simulink model "combined_model_withAC_2021b"  (R2021b)
settings: Solver=VariableStepAuto  StartTime=0.0  StopTime=5  RelTol=1e-3
model workspace (MAT data in the model file):
  C = 0.00044
  L = 0.00025
undefined symbols (not defined in the file): C_phi, Ls, poles, powergui, R_load, Rs, spspowerguiLib
libraries: spsDiodeLib x7, spsSeriesRLCBranchLib x6, spsVoltageMeasurementLib x5, spsMosfetLib x5, spsControlledVoltageSourceLib x3, simulink x3, spsCurrentMeasurementLib x2, spsParallelRLCBranchLib x2, spsGroundLib x1, spsParallelRLCLoadLib x1, spsVariableCapacitorLib x1
settings Model: Creator=maarten  LastModifiedBy=maarten
settings DebuggingCC: UnconnectedInputMsg=none  UnconnectedOutputMsg=none  UnconnectedLineMsg=none
settings ModelReferenceCC: EnableRefExpFcnMdlSchedulingChecks=off
settings RTWCC: DLArmComputeVersion=20.02.1

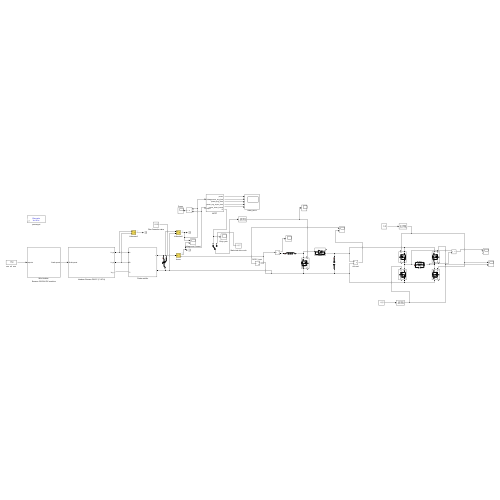
[thumbnail: Simulink's stored preview of the top-level diagram]
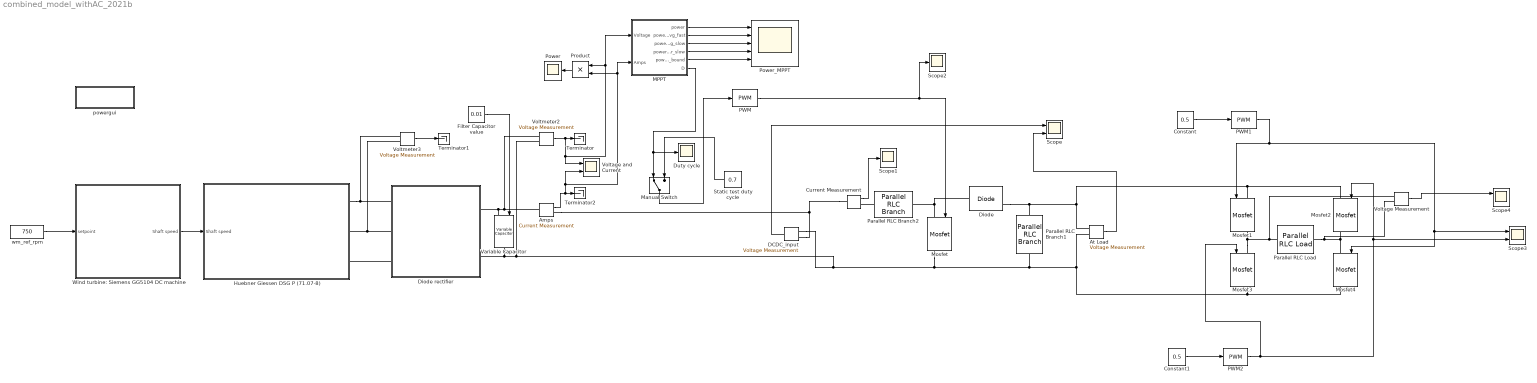
== system combined_model_withAC_2021b ==
  Amps : spsCurrentMeasurementLib/Current Measurement  PhasorSimulation=off  OutputType=Complex  PSBequivalent=0
  At Load : spsVoltageMeasurementLib/Voltage Measurement  PhasorSimulation=off  OutputType=Complex  PSBequivalent=0
  Constant : Constant  Value=0.5
  Constant1 : Constant  Value=0.5
  Current Measurement : spsCurrentMeasurementLib/Current Measurement  PhasorSimulation=off  OutputType=Complex  PSBequivalent=0
  DCDC_input : spsVoltageMeasurementLib/Voltage Measurement  PhasorSimulation=off  OutputType=Complex  PSBequivalent=0
  Diode : spsDiodeLib/Diode  Ron=0.001  Lon=0  Vf=0.8  IC=0  UseSnubber=0  Rs=500  Cs=250e-9  Measurements=on
  Diode rectifier : Subsystem
  Duty cycle : Scope
  Filter Capacitor value : Constant  Value=0.01
  "Huebner Giessen DSG P (71.07-8) " : Subsystem
  MPPT : Subsystem
  Manual Switch : ManualSwitch
  Mosfet{,1..4} (5 alike) : spsMosfetLib/Mosfet  Ron=0.1  Lon=0  Rd=0.01  Vfd=0  IC=0  Rs=1e5  Cs=inf  Measurements=on
  PWM : simulink/Discontinuities/PWM  DisableCoverage=on  Period=0.0001  InitialDelay=0  DisallowZeroDutyCycle=off  RunAtFixedTimeIntervals=off  SampleTime=0.1
  PWM1 : simulink/Discontinuities/PWM  DisableCoverage=on  Period=0.0005  InitialDelay=0  DisallowZeroDutyCycle=off  RunAtFixedTimeIntervals=off  SampleTime=0.1
  PWM2 : simulink/Discontinuities/PWM  DisableCoverage=on  Period=0.0005  InitialDelay=0.0005/2  DisallowZeroDutyCycle=off  RunAtFixedTimeIntervals=off  SampleTime=0.1
  Parallel RLC Branch1 : spsParallelRLCBranchLib/Parallel RLC Branch  LConnTagsString=a  RConnTagsString=__new0  BranchType=C  Resistance=R_load  Inductance=1e-3  SetiL0=off  InitialCurrent=0  Capacitance=C  Setx0=off  InitialVoltage=0  Measurements=None
  Parallel RLC Branch2 : spsParallelRLCBranchLib/Parallel RLC Branch  LConnTagsString=a  RConnTagsString=__new0  BranchType=L  Resistance=R_load  Inductance=L  SetiL0=off  InitialCurrent=0  Capacitance=C  Setx0=off  InitialVoltage=0  Measurements=None
  Parallel RLC Load : spsParallelRLCLoadLib/Parallel RLC Load  LConnTagsString=a  RConnTagsString=__new0  NominalVoltage=1000  NominalFrequency=60  ActivePower=10e3  InductivePower=100  CapacitivePower=100  Setx0=off  InitialVoltage=0  SetiL0=off  InitialCurrent=0  Measurements=None  LoadType=constant Z
      settings: AttributesFormatString=\n
  Power : Scope
  Power_MPPT : Scope  NumInputPorts=5
  Product : Product
  Scope : Scope  NumInputPorts=2
  Scope1 : Scope
  Scope2 : Scope
  Scope3 : Scope  NumInputPorts=2
  Scope4 : Scope  NumInputPorts=2
  Static test duty cycle : Constant  Value=0.7
  Terminator : Terminator
  Terminator1 : Terminator
  Terminator2 : Terminator
  Variable Capacitor : spsVariableCapacitorLib/Variable Capacitor  methode=Backward Euler  Cabsmin=1e-9  Initialize=off  vC0=0  C0=1e-6  iC0=0
  Voltage Measurement : spsVoltageMeasurementLib/Voltage Measurement  PhasorSimulation=off  OutputType=Complex  PSBequivalent=0
  Voltage and Current : Scope  NumInputPorts=2
  Voltmeter2 : spsVoltageMeasurementLib/Voltage Measurement  PhasorSimulation=off  OutputType=Complex  PSBequivalent=0
  Voltmeter3 : spsVoltageMeasurementLib/Voltage Measurement  PhasorSimulation=off  OutputType=Complex  PSBequivalent=0
  "Wind turbine: Siemens GG5104 DC machine " : Subsystem
  powergui : Subsystem  Priority=1  AncestorBlock=spspowerguiLib/powergui  DialogController=POWERSYS.PowerSysDialog  InitFcn=powergui( 'InitFcn_Callback' , gcb , 0 , [ ] );  mask(PSB option menu block){SimulationMode=Discrete, SampleTime=1e-6, frequency=60, Iterations=50, frequencyindice=0, Pbase=100e6, ErrMax=1e-4, UnitsV=kV, UnitsW=MW, buscounter=0, FunctionMessages=off, echomessages=off, EnableUseOfTLC=off, CurrentSourceSwitches=off, DisableSnubberDevices=off, DisableRonSwitches=off, DisableVfSwitches=off, DisplayEquations=off, AutomaticDiscreteSolvers=off, SolverType=Tustin, Interpol=off, ExternalGateDelay=off, methode=off, Ts=0, x0status=blocks, SPID=off, SwTol=0, HookPort=off, NonlinearTolerance=1e-4, nMaxIteration=100, ContinueOnMaxIteration=off, RestoreLinks=warning, ResistiveCurrentMeasurement=off, Frange=[0:2:500], Ylog=off, Xlog=on, ShowGrid=off, save=off, variable=ZData, structure=0, ZoomFFT=off, StartTime=0.0, cycles=1, DisplayStyle=1, fundamental=60, FreqAxis=off, MaxFrequency=1000, frequencyindicesteady=1, RmsSteady=1, display=off}
      mask prompts: SimulationMode "Simulation type:"; SampleTime "Sample time (s):"; frequency "Frequency (Hz):"; Iterations "Max iterations"; frequencyindice "Frequency (Hz)"; Pbase "Base power (VA)"; ErrMax "PQ tolerance (pu)"; UnitsV "Voltage units"; UnitsW "Power units"; buscounter "Load flow bus counter"; FunctionMessages "Disable Specialized Power Systems warnings"; echomessages "Display Specialized Power Systems compilation messages"; EnableUseOfTLC "Use TLC file when in Accelerator Simulation Mode and for code generation"; CurrentSourceSwitches "Disable ideal switching"; DisableSnubberDevices "Disable snubbers in switching devices"; DisableRonSwitches "Disable Ron resistances in switching devices"; DisableVfSwitches "Disable forward voltages in switching devices"; DisplayEquations "Display circuit differential equations"; AutomaticDiscreteSolvers "Automatically handle Discrete solver and Advanced tab solver settings of blocks"; SolverType "Discrete solver"; Interpol "Interpolate switching events"; ExternalGateDelay "Use time-stamped gate signals"; methode "Store switching topologies"; Ts "Buffer size (MBytes):"; x0status "Start simulation with initial electrical states from:"; SPID "Use ideal switching devices"; SwTol "Switch tolerance"; HookPort "Allow multiple powergui blocks"; NonlinearTolerance "Solver tolerance"; nMaxIteration "Maximum number of iterations"; ContinueOnMaxIteration "Continue Simulation if maximum number of iterations is reached"; RestoreLinks "Restore disabled links of Simscape Power Systems ST blocks:"; ResistiveCurrentMeasurement "Use non ideal current measurement blocks (1e-4Ohm internal resistance)"; Frange "Frequency Range"; Ylog "Log impedance"; Xlog "log Frequency"; ShowGrid "grid"; save "Save Data To Workspace"; variable "Variable Name"; structure "Structure Name (PSBFFTSCOPE)"; ZoomFFT "ZoomFFT (PSBFFTSCOPE)"; StartTime "Start Time (PSBFFTSCOPE)"; cycles "Cycles (PSBFFTSCOPE)"; DisplayStyle "Display style (PSBFFTSCOPE)"; fundamental "Fundamental (PSBFFTSCOPE)"; FreqAxis "Frequency Axis (PSBFFTSCOPE)"; MaxFrequency "Max Frequency (PSBFFTSCOPE)"; frequencyindicesteady "Frequency indice (STEADYSTATE)"; RmsSteady "RMS display (STEADYSTATE)"; display "Display Results"
      mask help: Set simulation type, simulation parameters, and preferences.
      mask init:
      | dispMessage = '';
      | dispMessage = powergui('MaskInitialization',gcb,SimulationMode,SampleTime);
      settings: PreSaveFcn=powergui( 'PreSaveFcn_Callback' , gcb , [ ] , [ ] );  OpenFcn=sps_rtmsupport('OpenFcn',gcbh)
      mask Help: helpview(psbhelp)
      mask TypeOptions SimulationMode: Continuous | Discrete | Phasor | Discrete phasor
      mask Callback SimulationMode: powergui('SimulationType',[],[],gcb);
      mask TypeOptions UnitsV: V | kV
      mask TypeOptions UnitsW: W | kW | MW
      mask Callback CurrentSourceSwitches: powergui('SimulationType',[],[],gcb);
      mask Callback AutomaticDiscreteSolvers: powergui('SimulationType',[],[],gcb);
      mask TypeOptions SolverType: Tustin/Backward Euler (TBE) | Tustin | Backward Euler
      mask Callback SolverType: powergui('SimulationType',[],[],gcb);
      mask Callback Interpol: powergui('SimulationType',[],[],gcb);
      mask Callback ExternalGateDelay: powergui('SimulationType',[],[],gcb);
      mask Callback methode: powergui('SimulationType',[],[],gcb);
      mask TypeOptions x0status: blocks | steady | zero
      mask TypeOptions RestoreLinks: yes | warning | no
      mask Callback display: sps_rtmsupport('parametereditingmodes',gcbh) % Will be executed last in parameter callbacks to ensure mask enable consistency
      mask DialogControl SolverTab Prompt: Solver
      mask DialogControl AutoSolverNote Prompt: The Simulation type parameter is governed by Simulink. To access the Powergui solver settings, unselect auto (Automatic solver selection) solver in the Simulink solver options.
      mask DialogControl Apps Prompt: Apps
      mask DialogControl StateAnalyzer Prompt: Measurements and States Analyzer
      mask DialogControl StateAnalyzer Callback: powerStates(bdroot(gcb))
      mask DialogControl LineParameterCalculator Prompt: Line Parameter Calculator
      mask DialogControl LineParameterCalculator Callback:
      | close_system(gcb)
      | powerLineParameters
      mask DialogControl CableParameterCalculator Prompt: Cable Parameter Calculator
      mask DialogControl CableParameterCalculator Callback:
      | close_system(gcb)
      | powerCableParameters
      mask DialogControl LineDecoupler Prompt: Line Decoupler
      mask DialogControl LineDecoupler Tooltip: Click to replace selected Distributed Parameters Line blocks with Decoupling Line blocks
      mask DialogControl LineDecoupler Callback:
      | close_system(gcb);
      | DecouplingLineReplace(gcs)
      mask DialogControl LoadFlowAnalyzer Prompt: Load Flow Analyzer
      mask DialogControl LoadFlowAnalyzer Callback:
      | close_system(gcb)
      | powerLoadFlow
      mask DialogControl LoadFlowParameters Prompt: Load Flow Parameters
      mask DialogControl ImpedanceCalculator Prompt: Impedance Calculator
      mask DialogControl ImpedanceCalculator Callback:
      | close_system(gcb);
      | powerImpedance(bdroot(gcs));
      mask DialogControl FFTAnalyzer Prompt: FFT Analyzer
      mask DialogControl FFTAnalyzer Callback:
      | close_system(gcb)
      | power_fftscope(bdroot(gcb),gcb)
      mask DialogControl LinearSystemAnalyzer Prompt: Linear System Analyzer
      mask DialogControl LinearSystemAnalyzer Callback:
      | close_system(gcb)
      | power_ltiview(bdroot(gcb))
      mask DialogControl HysteresisDesigner Prompt: Hysteresis Designer
      mask DialogControl HysteresisDesigner Callback:
      | close_system(gcb)
      | powerHysteresis('hysteresis.mat')
      mask DialogControl BlockCustomizer Prompt: Block Customizer
      mask DialogControl BlockCustomizer Callback:
      | close_system(gcb);
      | power_customize;
      mask DialogControl ReportGenerator Prompt: Report Generator
      mask DialogControl ReportGenerator Callback:
      | close_system(gcb)
      | power_report(bdroot(gcb))
      mask DialogControl obsolete Prompt: ...
      mask DialogControl MachineInitialization Prompt: Machine Initialization
      mask DialogControl MachineInitialization Callback:
      | close_system(gcb)
      | powericon('machineInitTool',bdroot(gcb),gcb)
      mask DialogControl Preferences Prompt: Preferences
      mask DialogControl Solver Prompt: Solver
      mask DialogControl SolverDetails Prompt: Solver details for nonlinear elements
      mask Display: color('blue'),disp(dispMessage)
  wm_ref_rpm : Constant  Value=750
  wires:
  MPPT/2(power_avg_fast) -> Power_MPPT/2
  MPPT/6(D) -> Manual Switch/1, Duty cycle/1
  PWM/1 -> Mosfet/1, Scope2/1
  "Wind turbine: Siemens GG5104 DC machine "/1(Shaft speed) -> "Huebner Giessen DSG P (71.07-8) "/1(Shaft speed)
  wm_ref_rpm/1 -> "Wind turbine: Siemens GG5104 DC machine "/1(setpoint)
  Static test duty cycle/1 -> Manual Switch/2
  Filter Capacitor value/1 -> Variable Capacitor/1
  MPPT/5(power_lower_bound) -> Power_MPPT/5
  MPPT/3(power_avg_slow) -> Power_MPPT/3
  MPPT/4(power_avg_super_slow) -> Power_MPPT/4
  Product/1 -> Power/1
  MPPT/1(power) -> Power_MPPT/1
  Amps/1 -> Voltage and Current/2, Product/2, MPPT/2(Amps), Terminator2/1
  At Load/1 -> Scope/2
  Voltmeter3/1 -> Terminator1/1
  DCDC_input/1 -> Scope/1
  Voltmeter2/1 -> MPPT/1(Voltage), Product/1, Voltage and Current/1, Terminator/1
  Manual Switch/1 -> PWM/1
  Current Measurement/1 -> Scope1/1
  Voltage Measurement/1 -> Scope4/1
  Constant1/1 -> PWM2/1
  Constant/1 -> PWM1/1
  PWM2/1 -> Mosfet3/1, Scope3/2, Mosfet2/1
  PWM1/1 -> Scope3/1, Mosfet4/1, Mosfet1/1
  connections:
  Mosfet3/RConn1 -- Variable Capacitor/RConn1 -- Diode rectifier/RConn2 -- Voltmeter2/LConn2 -- DCDC_input/LConn2 -- Mosfet/RConn1 -- Parallel RLC Branch1/RConn1 -- At Load/LConn2 -- Mosfet4/RConn1
  Mosfet/LConn1 -- Diode/LConn1 -- Parallel RLC Branch2/RConn1
  Mosfet1/LConn1 -- Diode/RConn1 -- Parallel RLC Branch1/LConn1 -- At Load/LConn1 -- Mosfet2/LConn1
  Amps/LConn1 -- Diode rectifier/RConn1 -- Variable Capacitor/LConn1 -- Voltmeter2/LConn1
  Voltmeter3/LConn2 -- "Huebner Giessen DSG P (71.07-8) "/RConn2 -- Diode rectifier/LConn2
  Current Measurement/LConn1 -- DCDC_input/LConn1 -- Amps/RConn1
  Voltmeter3/LConn1 -- Diode rectifier/LConn1 -- "Huebner Giessen DSG P (71.07-8) "/RConn1
  Diode rectifier/LConn3 -- "Huebner Giessen DSG P (71.07-8) "/RConn3
  Parallel RLC Branch2/LConn1 -- Current Measurement/RConn1
  Parallel RLC Load/RConn1 -- Voltage Measurement/LConn2 -- Mosfet4/LConn1 -- Mosfet2/RConn1
  Mosfet3/LConn1 -- Voltage Measurement/LConn1 -- Parallel RLC Load/LConn1 -- Mosfet1/RConn1

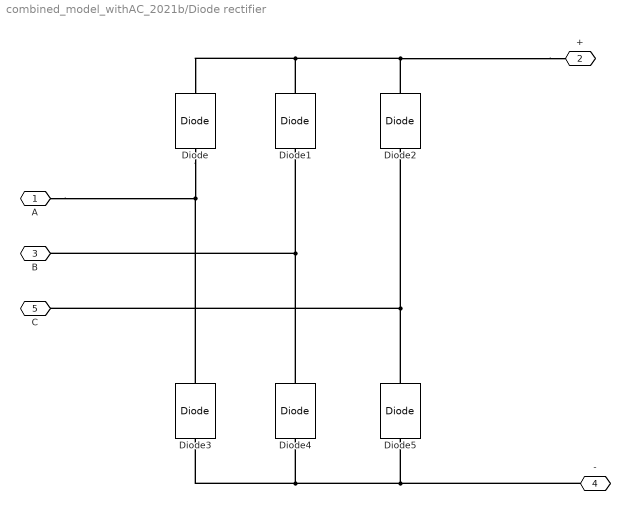
== system combined_model_withAC_2021b/Diode rectifier ==
  Diode{,1..5} (6 alike) : spsDiodeLib/Diode  Ron=0.01  Lon=0  Vf=0.85  IC=0  UseSnubber=off  Rs=500  Cs=250e-9  Measurements=off
  A : PMIOPort  Side=Left
  + : PMIOPort  Port=2  Side=Right
  B : PMIOPort  Port=3  Side=Left
  - : PMIOPort  Port=4  Side=Right
  C : PMIOPort  Port=5  Side=Left
  connections:
  Diode2/LConn1 -- C/RConn1 -- Diode5/RConn1
  +/RConn1 -- Diode2/RConn1 -- Diode1/RConn1 -- Diode/RConn1
  Diode3/LConn1 -- -/RConn1 -- Diode5/LConn1 -- Diode4/LConn1
  Diode3/RConn1 -- A/RConn1 -- Diode/LConn1
  Diode1/LConn1 -- B/RConn1 -- Diode4/RConn1

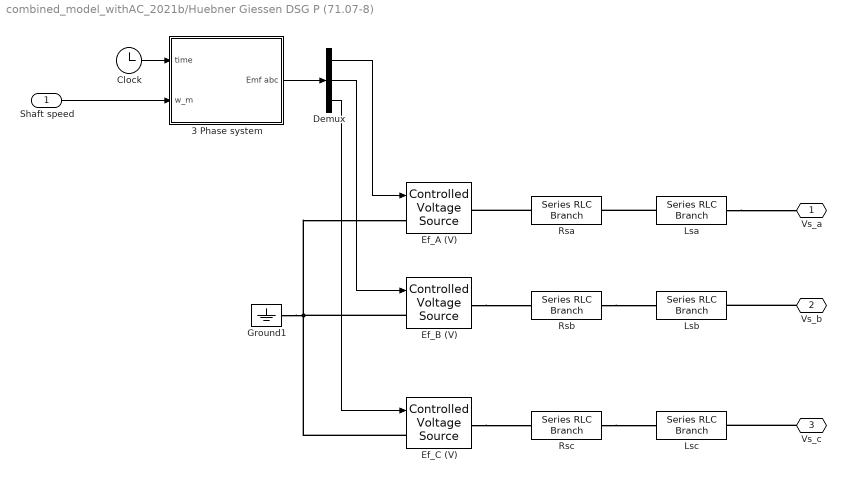
== system combined_model_withAC_2021b/Huebner Giessen DSG P (71.07-8)  ==
  Shaft speed : Inport
  "3 Phase system " : Subsystem
  Clock : Clock
  Demux : Demux  Outputs=3
  Ef_A (V) : spsControlledVoltageSourceLib/Controlled Voltage Source  Initialize=on  Source_Type=AC  Amplitude=0  Phase=0  Frequency=0  Measurements=None
  Ef_B (V) : spsControlledVoltageSourceLib/Controlled Voltage Source  Initialize=on  Source_Type=AC  Amplitude=0  Phase=0  Frequency=0  Measurements=None
  Ef_C (V) : spsControlledVoltageSourceLib/Controlled Voltage Source  Initialize=on  Source_Type=AC  Amplitude=0  Phase=0  Frequency=0  Measurements=None
  Ground1 : spsGroundLib/Ground  LConnTagsString=a
  Lsa : spsSeriesRLCBranchLib/Series RLC Branch  LConnTagsString=__new0  RConnTagsString=__new0  BranchType=L  Resistance=Rs  Inductance=Ls  SetiL0=off  InitialCurrent=0  Capacitance=1e-6  Setx0=off  InitialVoltage=0  Measurements=Branch current
  Lsb : spsSeriesRLCBranchLib/Series RLC Branch  LConnTagsString=__new0  RConnTagsString=__new0  BranchType=L  Resistance=Rs  Inductance=Ls  SetiL0=off  InitialCurrent=0  Capacitance=1e-6  Setx0=off  InitialVoltage=0  Measurements=Branch current
  Lsc : spsSeriesRLCBranchLib/Series RLC Branch  LConnTagsString=__new0  RConnTagsString=__new0  BranchType=L  Resistance=Rs  Inductance=Ls  SetiL0=on  InitialCurrent=0  Capacitance=1e-6  Setx0=off  InitialVoltage=0  Measurements=Branch current
  Rsa : spsSeriesRLCBranchLib/Series RLC Branch  LConnTagsString=__new0  RConnTagsString=__new0  BranchType=R  Resistance=Rs  Inductance=Ls  SetiL0=off  InitialCurrent=0  Capacitance=1e-6  Setx0=off  InitialVoltage=0  Measurements=Branch current
  Rsb : spsSeriesRLCBranchLib/Series RLC Branch  LConnTagsString=__new0  RConnTagsString=__new0  BranchType=R  Resistance=Rs  Inductance=Ls  SetiL0=off  InitialCurrent=0  Capacitance=1e-6  Setx0=off  InitialVoltage=0  Measurements=Branch current
  Rsc : spsSeriesRLCBranchLib/Series RLC Branch  LConnTagsString=__new0  RConnTagsString=__new0  BranchType=R  Resistance=Rs  Inductance=Ls  SetiL0=on  InitialCurrent=0  Capacitance=1e-6  Setx0=off  InitialVoltage=0  Measurements=Branch current
  Vs_a : PMIOPort  Side=Right
  Vs_b : PMIOPort  Port=2  Side=Right
  Vs_c : PMIOPort  Port=3  Side=Right
  wires:
  Demux/1 -> Ef_A (V)/1
  Demux/3 -> Ef_C (V)/1
  Demux/2 -> Ef_B (V)/1
  Shaft speed/1 -> "3 Phase system "/2(w_m)
  Clock/1 -> "3 Phase system "/1(time)
  "3 Phase system "/1("Emf abc ") -> Demux/1
  connections:
  Ef_B (V)/RConn1 -- Rsb/LConn1
  Lsa/RConn1 -- Vs_a/RConn1
  Vs_b/RConn1 -- Lsb/RConn1
  Ef_B (V)/LConn1 -- Ground1/LConn1 -- Ef_C (V)/LConn1 -- Ef_A (V)/LConn1
  Vs_c/RConn1 -- Lsc/RConn1
  Lsa/LConn1 -- Rsa/RConn1
  Ef_C (V)/RConn1 -- Rsc/LConn1
  Rsa/LConn1 -- Ef_A (V)/RConn1
  Rsb/RConn1 -- Lsb/LConn1
  Rsc/RConn1 -- Lsc/LConn1

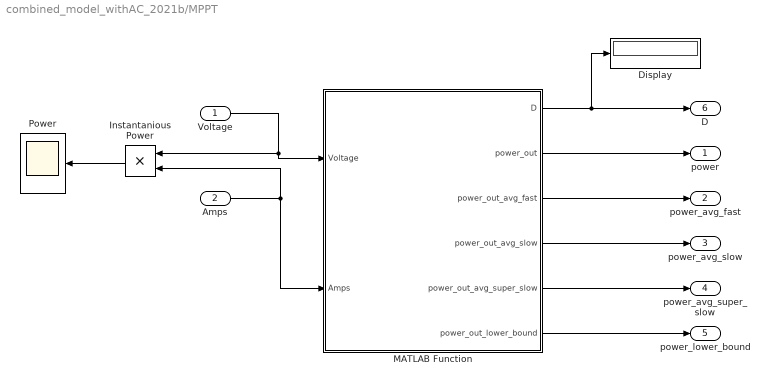
== system combined_model_withAC_2021b/MPPT ==
  Voltage : Inport
  Amps : Inport  Port=2
  Display : Display
  Instantanious Power : Product
  MATLAB Function : MATLAB Function  TreatAsAtomicUnit=on  SystemSampleTime=0.0002
  Power : Scope
  power : Outport
  power_avg_fast : Outport  Port=2
  power_avg_slow : Outport  Port=3
  power_avg_super_slow : Outport  Port=4
  power_lower_bound : Outport  Port=5
  D : Outport  Port=6
  wires:
  MATLAB Function/1(D) -> D/1, Display/1
  Instantanious Power/1 -> Power/1
  Voltage/1 -> Instantanious Power/1, MATLAB Function/1(Voltage)
  Amps/1 -> MATLAB Function/2(Amps), Instantanious Power/2
  MATLAB Function/2(power_out) -> power/1
  MATLAB Function/3(power_out_avg_fast) -> power_avg_fast/1
  MATLAB Function/4(power_out_avg_slow) -> power_avg_slow/1
  MATLAB Function/5(power_out_avg_super_slow) -> power_avg_super_slow/1
  MATLAB Function/6(power_out_lower_bound) -> power_lower_bound/1

== system combined_model_withAC_2021b/Wind turbine: Siemens GG5104 DC machine  ==
  setpoint : Inport
  Shaft speed : Outport
  wires:
  setpoint/1 -> Shaft speed/1

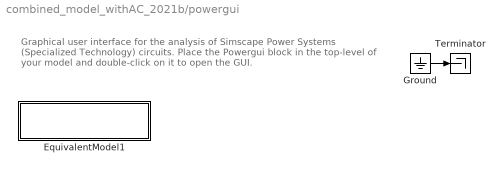
== system combined_model_withAC_2021b/powergui ==
  note: Graphical user interface for the analysis of
      | Simscape Power Systems (Specialized Technology) circuits.
      | Place the Powergui block in the top-level of your model and double-click
      | on it to open the GUI.
  EquivalentModel1 : Subsystem
      mask init:
      | S  = GetDataForEquivalentModel('Discrete',gcbh);
      mask Display: disp('EQUIVALENT CIRCUIT\nDSS')
  Ground : Ground
  Terminator : Terminator
  wires:
  Ground/1 -> Terminator/1

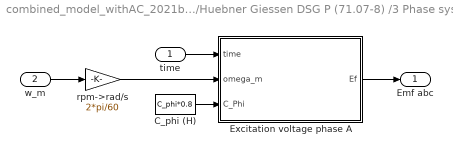
== system combined_model_withAC_2021b/Huebner Giessen DSG P (71.07-8) /3 Phase system  ==
  time : Inport
  w_m : Inport  Port=2
  C_phi (H) : Constant  Value=C_phi*0.8  VectorParams1D=off
  Excitation voltage phase A : Subsystem
  rpm->rad/s : Gain  Gain=2*pi/60
  "Emf abc " : Outport
  wires:
  w_m/1 -> rpm->rad/s/1
  C_phi (H)/1 -> Excitation voltage phase A/3(C_Phi)
  time/1 -> Excitation voltage phase A/1(time)
  rpm->rad/s/1 -> Excitation voltage phase A/2(omega_m)
  Excitation voltage phase A/1(Ef) -> "Emf abc "/1

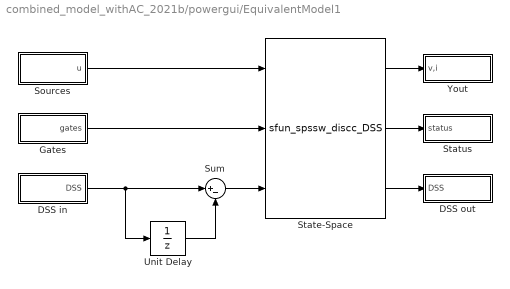
== system combined_model_withAC_2021b/powergui/EquivalentModel1 ==
  DSS in : Subsystem
  DSS out : Subsystem
  Gates : Subsystem
  Sources : Subsystem
  State-Space : S-Function  FunctionName=sfun_spssw_discc_DSS  Parameters="S.Ts, S.A, S.B, S.C, S.D, S.x0, S.EnableUseOfTLC, S.NonLinearDim,  S.NonLinearxInit, S.NonLinear_Inputs, S.NonLinear_Outputs, S.NonLinear_InitialOutputs, S.NonLinearIterative, S.NonLinear_SizeVI,  S.NonLinear_VI, S.NonLinear_Method , S.Nonlinear_Tolerance, double(nMaxIteration), double(ContinueOnMaxIteration),S.SwitchResistance ,S.SwitchType, S.SwitchGateInitialValue, S.OutputsToResetToZero, double(S.TBEON)"  SFunctionModules=DSS_Utils  SFunctionDeploymentMode=off  EnableBusSupport=off
  Status : Subsystem
  Sum : Sum  Inputs=|+-
  Unit Delay : UnitDelay  SampleTime=S.Ts  HasFrameUpgradeWarning=on
  Yout : Subsystem
  wires:
  Sum/1 -> State-Space/3
  Unit Delay/1 -> Sum/2
  DSS in/1(DSS) -> Sum/1, Unit Delay/1
  Gates/1(gates) -> State-Space/2
  Sources/1(u) -> State-Space/1
  State-Space/2 -> Status/1(status)
  State-Space/1 -> Yout/1(v,i)
  State-Space/3 -> DSS out/1(DSS)

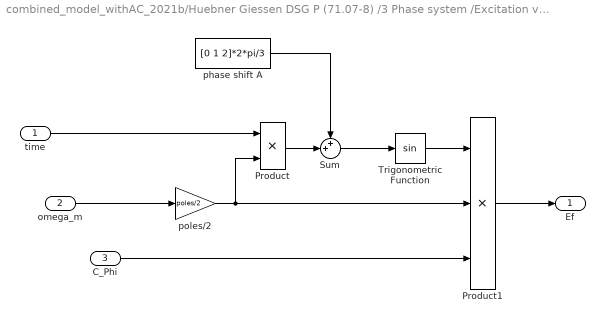
== system combined_model_withAC_2021b/Huebner Giessen DSG P (71.07-8) /3 Phase system /Excitation voltage phase A ==
  time : Inport
  omega_m : Inport  Port=2
  C_Phi : Inport  Port=3
  Product : Product  RndMeth=Zero
  Product1 : Product  Inputs=3  RndMeth=Zero
  Sum : Sum  Inputs=++|
  Trigonometric Function : Trigonometry
  phase shift A : Constant  Value=[0 1 2]*2*pi/3
  poles/2 : Gain  Gain=poles/2
  Ef : Outport
  wires:
  poles/2/1 -> Product/2, Product1/2
  Trigonometric Function/1 -> Product1/1
  phase shift A/1 -> Sum/1
  Product/1 -> Sum/2
  Product1/1 -> Ef/1
  C_Phi/1 -> Product1/3
  Sum/1 -> Trigonometric Function/1
  time/1 -> Product/1
  omega_m/1 -> poles/2/1

== system combined_model_withAC_2021b/powergui/EquivalentModel1/DSS in ==
  Mux : Mux  Inputs=1
  DSS : Outport  VectorParamsAs1DForOutWhenUnconnected=off
  wires:
  Mux/1 -> DSS/1
  [T58_5457_5876453571207] -> Mux/1

== system combined_model_withAC_2021b/powergui/EquivalentModel1/DSS out ==
  DSS : Inport
  Demux : Demux  Outputs=1
  Goto1 : Terminator
  wires:
  DSS/1 -> Demux/1
  Demux/1 -> Goto1/1

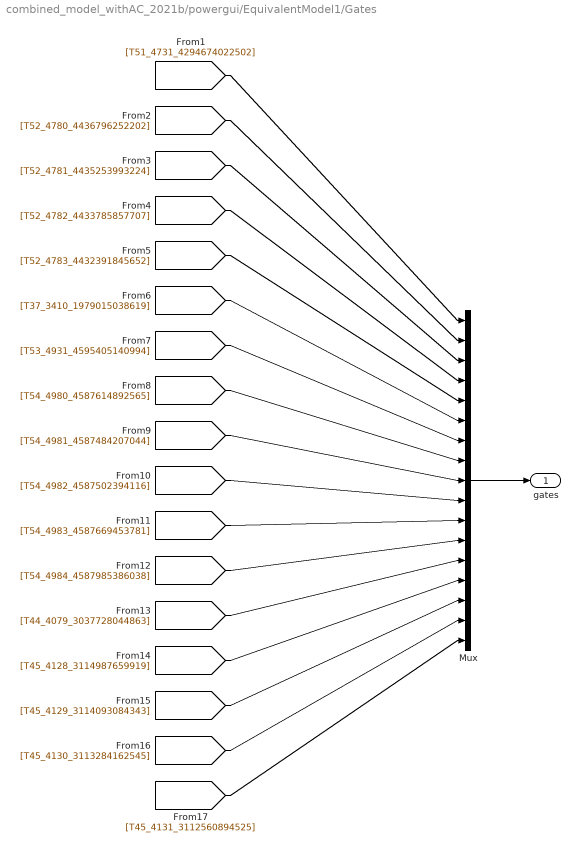
== system combined_model_withAC_2021b/powergui/EquivalentModel1/Gates ==
  Mux : Mux  Inputs=[1 1 1 1 1 1 1 1 1 1 1 1 1 1 1 1 1]
  gates : Outport  VectorParamsAs1DForOutWhenUnconnected=off
  wires:
  Mux/1 -> gates/1
  [T51_4731_4294674022502] -> Mux/1
  [T52_4780_4436796252202] -> Mux/2
  [T52_4781_4435253993224] -> Mux/3
  [T52_4782_4433785857707] -> Mux/4
  [T52_4783_4432391845652] -> Mux/5
  [T37_3410_1979015038619] -> Mux/6
  [T53_4931_4595405140994] -> Mux/7
  [T54_4980_4587614892565] -> Mux/8
  [T54_4981_4587484207044] -> Mux/9
  [T54_4982_4587502394116] -> Mux/10
  [T54_4983_4587669453781] -> Mux/11
  [T54_4984_4587985386038] -> Mux/12
  [T44_4079_3037728044863] -> Mux/13
  [T45_4128_3114987659919] -> Mux/14
  [T45_4129_3114093084343] -> Mux/15
  [T45_4130_3113284162545] -> Mux/16
  [T45_4131_3112560894525] -> Mux/17

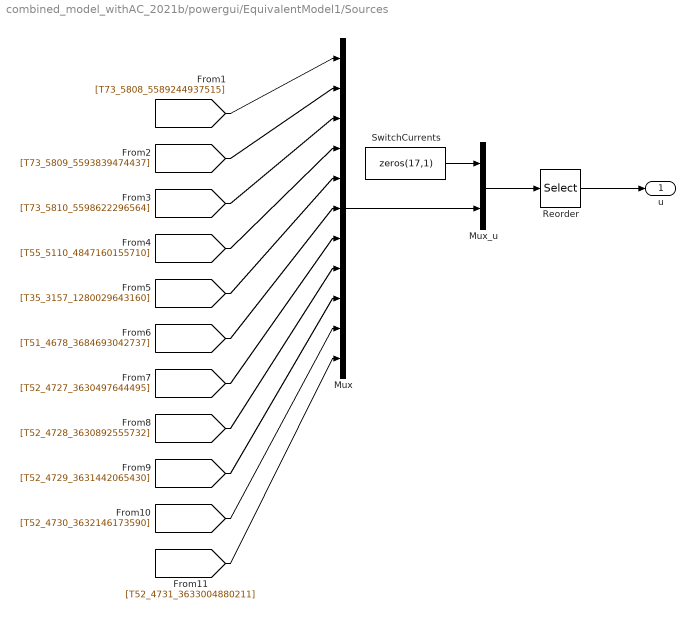
== system combined_model_withAC_2021b/powergui/EquivalentModel1/Sources ==
  Mux : Mux  Inputs=[1 1 1 1 1 1 1 1 1 1 1]
  Mux_u : Mux  Inputs=[17 11]
  Reorder : Selector  InputPortWidth=28  IndexOptions=Index vector (dialog)  Indices=[1 2 3 4 5 6 7 8 9 10 11 12 13 14 15 16 17 18 19 20 22 23 24 25 26 27 28 21]  OutputSizes=1
  SwitchCurrents : Constant  Value=zeros(17,1)
  u : Outport  VectorParamsAs1DForOutWhenUnconnected=off
  wires:
  Mux_u/1 -> Reorder/1
  SwitchCurrents/1 -> Mux_u/1
  Mux/1 -> Mux_u/2
  Reorder/1 -> u/1
  [T73_5808_5589244937515] -> Mux/1
  [T73_5809_5593839474437] -> Mux/2
  [T73_5810_5598622296564] -> Mux/3
  [T55_5110_4847160155710] -> Mux/4
  [T35_3157_1280029643160] -> Mux/5
  [T51_4678_3684693042737] -> Mux/6
  [T52_4727_3630497644495] -> Mux/7
  [T52_4728_3630892555732] -> Mux/8
  [T52_4729_3631442065430] -> Mux/9
  [T52_4730_3632146173590] -> Mux/10
  [T52_4731_3633004880211] -> Mux/11

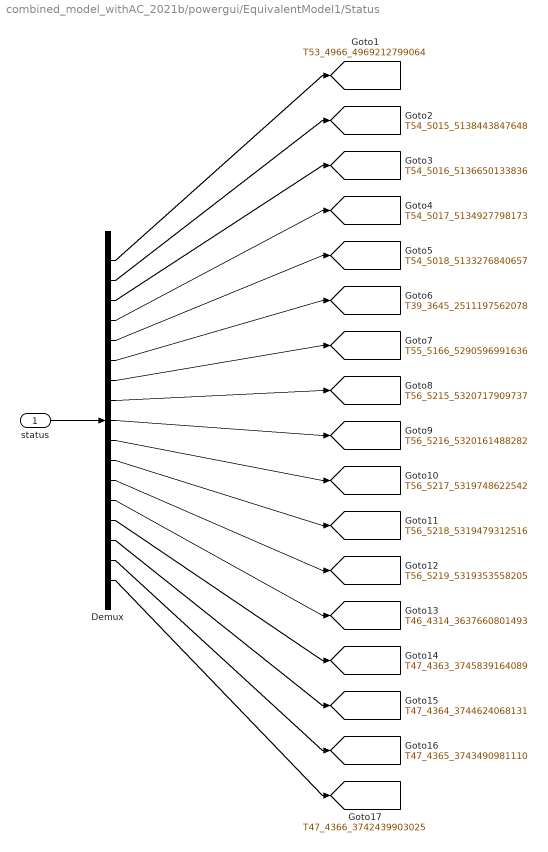
== system combined_model_withAC_2021b/powergui/EquivalentModel1/Status ==
  status : Inport
  Demux : Demux  Outputs=[1 1 1 1 1 1 1 1 1 1 1 1 1 1 1 1 1]
  tag scope: T39_3645_2511197562078=global, T46_4314_3637660801493=global, T47_4363_3745839164089=global, T47_4364_3744624068131=global, T47_4365_3743490981110=global, T47_4366_3742439903025=global, T53_4966_4969212799064=global, T54_5015_5138443847648=global, T54_5016_5136650133836=global, T54_5017_5134927798173=global, T54_5018_5133276840657=global, T55_5166_5290596991636=global, T56_5215_5320717909737=global, T56_5216_5320161488282=global, T56_5217_5319748622542=global, T56_5218_5319479312516=global, T56_5219_5319353558205=global
  wires:
  status/1 -> Demux/1
  Demux/1 -> [T53_4966_4969212799064]
  Demux/2 -> [T54_5015_5138443847648]
  Demux/3 -> [T54_5016_5136650133836]
  Demux/4 -> [T54_5017_5134927798173]
  Demux/5 -> [T54_5018_5133276840657]
  Demux/6 -> [T39_3645_2511197562078]
  Demux/7 -> [T55_5166_5290596991636]
  Demux/8 -> [T56_5215_5320717909737]
  Demux/9 -> [T56_5216_5320161488282]
  Demux/10 -> [T56_5217_5319748622542]
  Demux/11 -> [T56_5218_5319479312516]
  Demux/12 -> [T56_5219_5319353558205]
  Demux/13 -> [T46_4314_3637660801493]
  Demux/14 -> [T47_4363_3745839164089]
  Demux/15 -> [T47_4364_3744624068131]
  Demux/16 -> [T47_4365_3743490981110]
  Demux/17 -> [T47_4366_3742439903025]

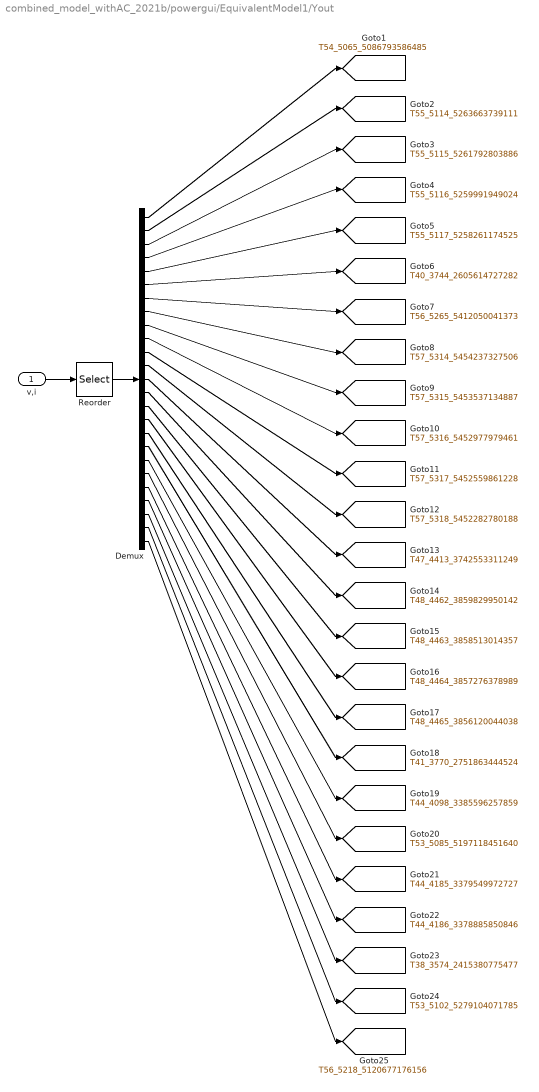
== system combined_model_withAC_2021b/powergui/EquivalentModel1/Yout ==
  v,i : Inport
  Demux : Demux  Outputs=[1 1 1 1 1 1 1 1 1 1 1 1 1 1 1 1 1 1 1 1 1 1 1 1 1]
  Reorder : Selector  InputPortWidth=25  IndexOptions=Index vector (dialog)  Indices=[1 2 3 4 5 6 7 8 9 10 11 12 13 14 15 16 17 18 19 20 21 22 23 24 25]  OutputSizes=1
  tag scope: T38_3574_2415380775477=global, T40_3744_2605614727282=global, T41_3770_2751863444524=global, T44_4098_3385596257859=global, T44_4185_3379549972727=global, T44_4186_3378885850846=global, T47_4413_3742553311249=global, T48_4462_3859829950142=global, T48_4463_3858513014357=global, T48_4464_3857276378989=global, T48_4465_3856120044038=global, T53_5085_5197118451640=global, T53_5102_5279104071785=global, T54_5065_5086793586485=global, T55_5114_5263663739111=global, T55_5115_5261792803886=global, T55_5116_5259991949024=global, T55_5117_5258261174525=global, T56_5218_5120677176156=global, T56_5265_5412050041373=global, T57_5314_5454237327506=global, T57_5315_5453537134887=global, T57_5316_5452977979461=global, T57_5317_5452559861228=global, T57_5318_5452282780188=global
  wires:
  v,i/1 -> Reorder/1
  Reorder/1 -> Demux/1
  Demux/1 -> [T54_5065_5086793586485]
  Demux/2 -> [T55_5114_5263663739111]
  Demux/3 -> [T55_5115_5261792803886]
  Demux/4 -> [T55_5116_5259991949024]
  Demux/5 -> [T55_5117_5258261174525]
  Demux/6 -> [T40_3744_2605614727282]
  Demux/7 -> [T56_5265_5412050041373]
  Demux/8 -> [T57_5314_5454237327506]
  Demux/9 -> [T57_5315_5453537134887]
  Demux/10 -> [T57_5316_5452977979461]
  Demux/11 -> [T57_5317_5452559861228]
  Demux/12 -> [T57_5318_5452282780188]
  Demux/13 -> [T47_4413_3742553311249]
  Demux/14 -> [T48_4462_3859829950142]
  Demux/15 -> [T48_4463_3858513014357]
  Demux/16 -> [T48_4464_3857276378989]
  Demux/17 -> [T48_4465_3856120044038]
  Demux/18 -> [T41_3770_2751863444524]
  Demux/19 -> [T44_4098_3385596257859]
  Demux/20 -> [T53_5085_5197118451640]
  Demux/21 -> [T44_4185_3379549972727]
  Demux/22 -> [T44_4186_3378885850846]
  Demux/23 -> [T38_3574_2415380775477]
  Demux/24 -> [T53_5102_5279104071785]
  Demux/25 -> [T56_5218_5120677176156]

== matlab function combined_model_withAC_2021b/MPPT/MATLAB Function ==
  settings: updateMethod=DISCRETE
  data: Voltage input double; Amps input double; D output double; power_out output double; power_out_avg_fast output; power_out_avg_slow output; power_out_avg_super_slow output; power_out_lower_bound output
function [D, power_out, power_out_avg_fast, power_out_avg_slow, power_out_avg_super_slow, power_out_lower_bound] = fcn(Voltage, Amps)

persistent timeout D_previous direction_previous fast_power_average super_slow_power_average slow_power_average power_lower_bound slow_power_array super_slow_power_array fast_power_array setfast setslow; %counter power_previous 
step_size = 0.0005;
super_slow_filter_size = 5000;
slow_filter_size = 500;
fast_filter_size = 100;
lower_bound_value = 0.95;


if isempty(D_previous)
    setfast = 0;
    timeout = 0;
    setslow = 0;
    D_previous = 0.9;
    direction_previous = 0;
    super_slow_power_array = zeros(super_slow_filter_size,1);
    slow_power_array = zeros(slow_filter_size,1);
    fast_power_array = zeros(fast_filter_size,1);
end

super_slow_power_array(2:end) = super_slow_power_array(1:end-1);
slow_power_array(2:end) = slow_power_array(1:end-1);
fast_power_array(2:end) = fast_power_array(1:end-1);



power = Voltage * Amps;
super_slow_power_array(1) = power;
slow_power_array(1) = power;
fast_power_array(1) = power;

super_slow_power_average = mean(super_slow_power_array);
slow_power_average = mean(slow_power_array);
fast_power_average = mean(fast_power_array);
power_lower_bound = lower_bound_value * super_slow_power_average;
direction = direction_previous;

if slow_power_average > fast_power_average && setfast == 0
    setfast = 1;
    if direction_previous == 1
        direction = 0;
    else
        direction = 1;
    end
end

if power_lower_bound < fast_power_average
    timeout = timeout + 1;
end

%if power_lower_bound > fast_power_average && setslow == 0 && timeout > 100
%    setslow = 1;
%    timeout = 0;
%    if direction_previous == 1
%        direction = 0;
%    else
%        direction = 1;
%    end
%end

if power_lower_bound < fast_power_average
    setslow = 0;
end

if slow_power_average < fast_power_average
    setfast = 0;
end

D = D_previous + (1.213-D_previous) * ((step_size * direction) - (step_size * (1 - direction)));

D_previous = D;
power_out_avg_slow = slow_power_average;
power_out = power;
power_out_avg_fast = fast_power_average;
power_out_avg_super_slow = super_slow_power_average;
power_out_lower_bound = power_lower_bound;
direction_previous = direction;
